simulink model "WindowFunction_Ex2"  (R2023a)
settings: Solver=VariableStepAuto  StartTime=0.0  StopTime=0.2  RelTol=1e-3
undefined symbols (not defined in the file): S, vsva2197, xcvc1902
libraries: dspsrcs4 x2, aieDSP x1, dspsigops x1, vmcUtilities x1
settings Model: Creator=sdegala  LastModifiedBy=robg
settings ModelReferenceCC: EnableRefExpFcnMdlSchedulingChecks=on

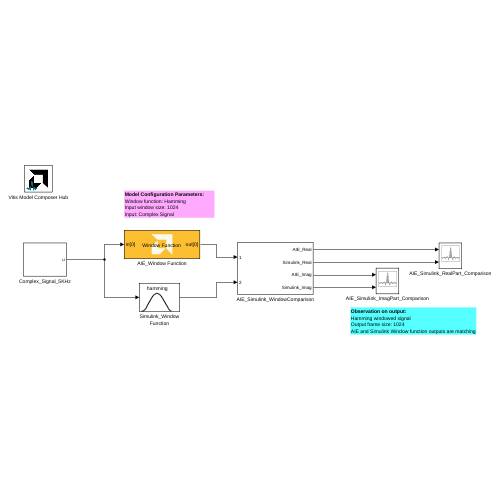
[thumbnail: Simulink's stored preview of the top-level diagram]
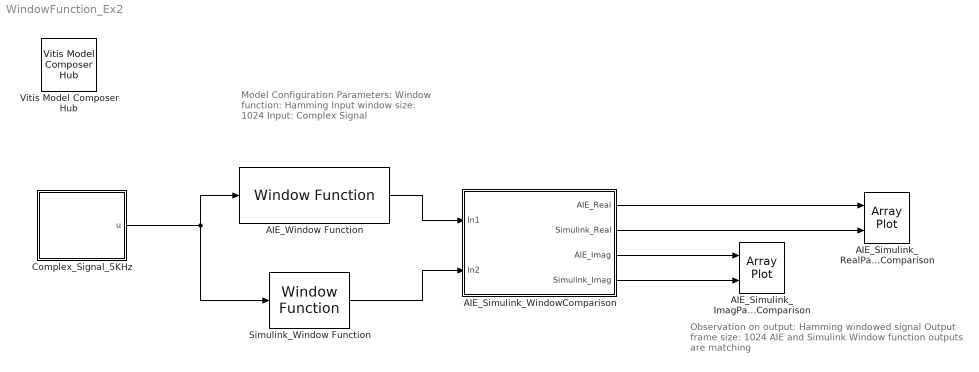
== system WindowFunction_Ex2 ==
  note: Model Configuration Parameters:
      | Window function: Hamming
      | Input window size: 1024
      | Input: Complex Signal
  note: Observation on output:
      | Hamming windowed signal
      | Output frame size: 1024
      | AIE and Simulink Window function outputs are matching
  AIE_Simulink_ImagPart_Comparison : ArrayPlot  NumInputPorts=2  WindowPosition=[240.000000,110.000000,800.000000,500.000000,]  PlotType=Line  AxesScaling=Manual  YLimits=[-5,5]  ShowLegend=on
  AIE_Simulink_RealPart_Comparison : ArrayPlot  NumInputPorts=2  WindowPosition=[5.000000,41.000000,1272.000000,651.000000,]  PlotType=Line  YLimits=[-1.2886,1.2856]  ShowLegend=on
  AIE_Simulink_WindowComparison : Subsystem
  AIE_Window Function : aieDSP/Window Function  data_type=cfloat  coeff_type=float  coeff=hamming(1024)  point_size=1024  is_dyn_pt_size=off  input_window_size=1024  shift_val=0  AIE_VARIANT=1  blockJsonConstraints=[]  blockJsonConstraintsInternal=[]  spec=vmc_fft_window.json  SerializedMaskParamNames=[]  SerializedMaskParamValues=[]  SerializedMaskParamVisibilities=[]  block_type=Window Function  SerializedMaskParamDataypes=typename|typename|coeff_type|uint|bool|uint|uint|uint  SerializedMaskParamEnumStrArr=0|0|0|0|0|0|0|0  SerializedMaskParamEnumValArr=0|0|0|0|0|0|0|0  SerializedMaskParamVectorArr=0|0|1|0|0|0|0|0
  Complex_Signal_5KHz : Subsystem
  Simulink_Window Function : dspsigops/Window Function  winmode=Apply window to input  wintype=Hamming  sampmode=Discrete  samptime=1  N=64  Rs=50  beta=10  winsamp=Periodic  UserWindow=hamming  OptParams=off  UserParams={'symmetric'}  dataType=double  isSigned=on  wordLen=16  udDataType=sfix(16)  fracBitsMode=Best precision  numFracBits=15  roundingMode=Round  overflowMode=off  numSidelobes=4  sidelobeLevel=-30
  Vitis Model Composer Hub : vmcUtilities/Vitis Model Composer Hub  Tag=genX  CodeGeneration=off  StartColumn=1  NumberOfColumns=1  TargetDirectory=./code  exportDesign=off  analyzeDesign=off  validateDesignOnHw=off  ExportType=AI Engines  IpVendor=xilinx.com  IpLibrary=hls  IpVersion=1.0  IpHWLanguage=Verilog  AieCompilerOptions={}  AieSimulatorOptions={}  CreateTestbench=off  TestbenchStackSize=10  RunRtlSim=off  RunCSim=off  RunAieSim=off  AieSimTimeout=50000  RunAieSimProfiling=off  LaunchVitisAnalyzer=off  PlotOutput=off  RunX86Sim=off  X86SimTimeout=10  GenHwImage=off  GenLibadfXo=off  GenHwValidationCode=off  PlatformType=Not Specified  HwSystemType=Baremetal  HwValidationTarget=hw  ProjDevice=xcvc1902-vsva2197-1LP-e-S  ProjDevicePart=xcvc1902-vsva2197-1LP-e-S  AIEType=AIE  SamplePeriod=-1  ClockFrequency=200  DataPathParallelism=1  xilinxfamily=versalaicore  part=xcvc1902  speed=-1LP-e-S  package=vsva2197  directory=./netlist  testbench=off  incr_netlist=off  synthesis_tool=Vivado  clock_wrapper=Clock Enables  dbl_ovrd=According to Block Masks  dcm_input_clock_period=10  sysclk_period=10  simulink_period=1  eval_field=0  LogFileName=''  NThreads=4
  wires:
  Complex_Signal_5KHz/1(u) -> AIE_Window Function/1, Simulink_Window Function/1
  AIE_Simulink_WindowComparison/1(AIE_Real) -> AIE_Simulink_RealPart_Comparison/1
  AIE_Simulink_WindowComparison/3(AIE_Imag) -> AIE_Simulink_ImagPart_Comparison/1
  AIE_Simulink_WindowComparison/4(Simulink_Imag) -> AIE_Simulink_ImagPart_Comparison/2
  AIE_Window Function/1 -> AIE_Simulink_WindowComparison/1(In1)
  Simulink_Window Function/1 -> AIE_Simulink_WindowComparison/2(In2)
  AIE_Simulink_WindowComparison/2(Simulink_Real) -> AIE_Simulink_RealPart_Comparison/2

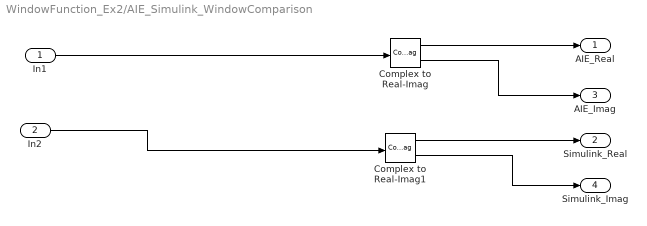
== system WindowFunction_Ex2/AIE_Simulink_WindowComparison ==
  In1 : Inport
  In2 : Inport  Port=2
  Complex to Real-Imag : ComplexToRealImag
  Complex to Real-Imag1 : ComplexToRealImag
  AIE_Real : Outport
  Simulink_Real : Outport  Port=2
  AIE_Imag : Outport  Port=3
  Simulink_Imag : Outport  Port=4
  wires:
  Complex to Real-Imag1/2 -> Simulink_Imag/1
  Complex to Real-Imag1/1 -> Simulink_Real/1
  In1/1 -> Complex to Real-Imag/1
  In2/1 -> Complex to Real-Imag1/1
  Complex to Real-Imag/1 -> AIE_Real/1
  Complex to Real-Imag/2 -> AIE_Imag/1

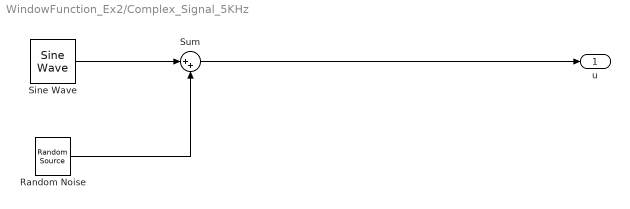
== system WindowFunction_Ex2/Complex_Signal_5KHz ==
  Random Noise : dspsrcs4/Random Source  SrcType=Gaussian  NormMethod=Ziggurat  CltLength=12  MinVal=0  MaxVal=1  MeanVal=0  VarVal=1e-3  RepMode=Not repeatable  rawSeed=1  IsInherit=off  SampMode=Discrete  SampTime=1/50e3  SampFrame=1024  DataType=Single  OutComplex=Real  OutputFrames=off
  Sine Wave : dspsrcs4/Sine Wave  Amplitude=1  Frequency=5e3  Phase=0  SampleMode=Discrete  OutComplex=Complex  CompMethod=Trigonometric fcn  TableSize=Speed  SampleTime=1/50e3  SamplesPerFrame=1024  ResetState=Restart at time zero  OutputFrames=off  dataType=single  wordLen=16  udDataType=sfix(16)  fracBitsMode=Best precision  numFracBits=15  OutDataTypeStr=single  LastOutDataTypeStr=single
  Sum : Sum  Inputs=|++
  u : Outport
  wires:
  Sine Wave/1 -> Sum/1
  Random Noise/1 -> Sum/2
  Sum/1 -> u/1
